simulink model "kalman"  (R2018b)
settings: Solver=VariableStepAuto  StartTime=0.0  StopTime=10.0  RelTol=1e-3
settings Model: Creator=axelwillekens  LastModifiedBy=axelwillekens

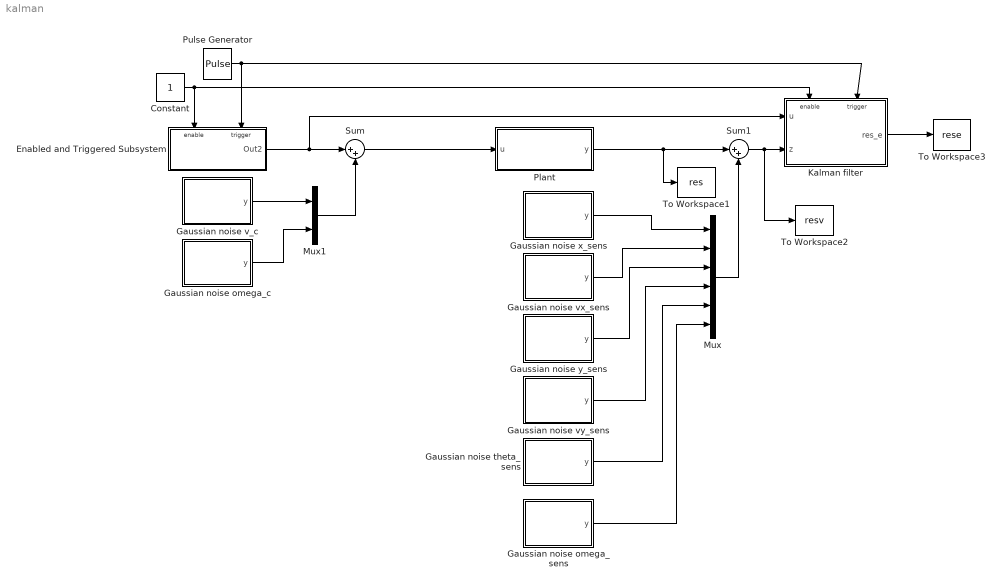
== system kalman ==
  Constant : Constant
  Enabled and Triggered Subsystem : Subsystem  TreatAsAtomicUnit=on
  Gaussian noise omega_c : MATLAB Function  TreatAsAtomicUnit=on
  Gaussian noise omega_sens : MATLAB Function  TreatAsAtomicUnit=on
  Gaussian noise theta_sens : MATLAB Function  TreatAsAtomicUnit=on
  Gaussian noise v_c : MATLAB Function  TreatAsAtomicUnit=on
  Gaussian noise vx_sens : MATLAB Function  TreatAsAtomicUnit=on
  Gaussian noise vy_sens : MATLAB Function  TreatAsAtomicUnit=on
  Gaussian noise x_sens : MATLAB Function  TreatAsAtomicUnit=on
  Gaussian noise y_sens : MATLAB Function  TreatAsAtomicUnit=on
  Kalman filter : Subsystem  TreatAsAtomicUnit=on
  Mux : Mux  Inputs=6
  Mux1 : Mux  Inputs=2
  Plant : Subsystem
  Pulse Generator : DiscretePulseGenerator  PulseType=Time based  Period=0.05  PulseWidth=5
  Sum : Sum  Inputs=|++
  Sum1 : Sum  Inputs=|++
  To Workspace1 : ToWorkspace  VariableName=res  SaveFormat=Timeseries  SampleTime=-1
  To Workspace2 : ToWorkspace  VariableName=resv  SaveFormat=Timeseries  SampleTime=-1
  To Workspace3 : ToWorkspace  VariableName=rese  SaveFormat=Timeseries  SampleTime=-1
  wires:
  Sum/1 -> Plant/1(u)
  Plant/1(y) -> To Workspace1/1, Sum1/1
  Sum1/1 -> To Workspace2/1, Kalman filter/2(z)
  Mux/1 -> Sum1/2
  Gaussian noise x_sens/1(y) -> Mux/1
  Gaussian noise vx_sens/1(y) -> Mux/2
  Gaussian noise y_sens/1(y) -> Mux/3
  Gaussian noise vy_sens/1(y) -> Mux/4
  Gaussian noise theta_sens/1(y) -> Mux/5
  Gaussian noise omega_sens/1(y) -> Mux/6
  Mux1/1 -> Sum/2
  Gaussian noise v_c/1(y) -> Mux1/1
  Gaussian noise omega_c/1(y) -> Mux1/2
  Enabled and Triggered Subsystem/1(Out2) -> Kalman filter/1(u), Sum/1
  Constant/1 -> Kalman filter/Enable, Enabled and Triggered Subsystem/Enable
  Pulse Generator/1 -> Enabled and Triggered Subsystem/Trigger, Kalman filter/Trigger
  Kalman filter/1(res_e) -> To Workspace3/1

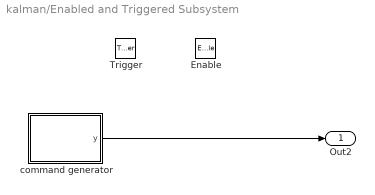
== system kalman/Enabled and Triggered Subsystem ==
  Enable : EnablePort
  Trigger : TriggerPort  VariantControl=Variant
  command generator : MATLAB Function  TreatAsAtomicUnit=on
  Out2 : Outport
  wires:
  command generator/1(y) -> Out2/1

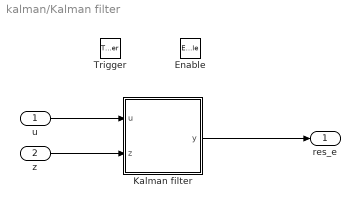
== system kalman/Kalman filter ==
  u : Inport
  z : Inport  Port=2
  Enable : EnablePort
  Trigger : TriggerPort  VariantControl=Variant
  Kalman filter : MATLAB Function  TreatAsAtomicUnit=on
  res_e : Outport
  wires:
  Kalman filter/1(y) -> res_e/1
  u/1 -> Kalman filter/1(u)
  z/1 -> Kalman filter/2(z)

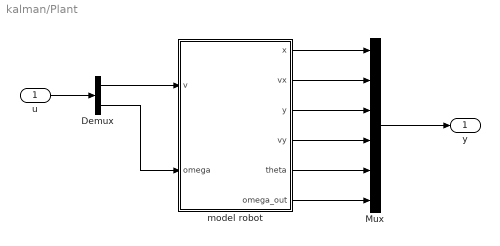
== system kalman/Plant ==
  u : Inport
  Demux : Demux  Outputs=2
  Mux : Mux  Inputs=6
  model robot : Subsystem
  y : Outport
  wires:
  Demux/1 -> model robot/1(v)
  Demux/2 -> model robot/2(omega)
  u/1 -> Demux/1
  model robot/1(x) -> Mux/1
  model robot/2(vx) -> Mux/2
  model robot/3(y) -> Mux/3
  model robot/4(vy) -> Mux/4
  model robot/5(theta) -> Mux/5
  model robot/6(omega_out) -> Mux/6
  Mux/1 -> y/1

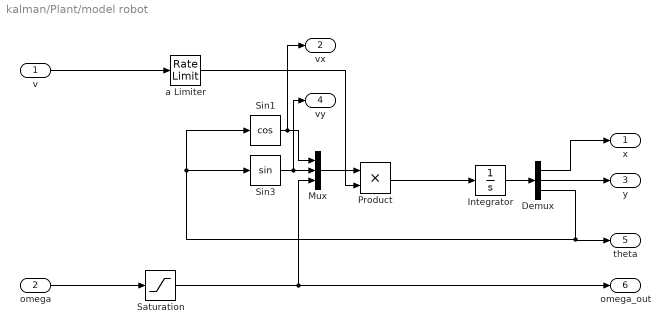
== system kalman/Plant/model robot ==
  v : Inport
  omega : Inport  Port=2
  Demux : Demux  Outputs=3
  Integrator : Integrator  InitialCondition=[2 -1 pi]
  Mux : Mux  Inputs=3
  Product : Product
  Saturation : Saturate  UpperLimit=50*(pi/180)  LowerLimit=-50*(pi/180)
  Sin1 : Trigonometry  Operator=cos
  Sin3 : Trigonometry
  a Limiter : RateLimiter  SampleTimeMode=inherited
  x : Outport
  vx : Outport  Port=2
  y : Outport  Port=3
  vy : Outport  Port=4
  theta : Outport  Port=5
  omega_out : Outport  Port=6
  wires:
  a Limiter/1 -> Product/2
  Mux/1 -> Product/1
  Product/1 -> Integrator/1
  Integrator/1 -> Demux/1
  Demux/2 -> y/1
  Demux/1 -> x/1
  Demux/3 -> Sin3/1, Sin1/1, theta/1
  Sin1/1 -> vx/1, Mux/1
  omega/1 -> Saturation/1
  Sin3/1 -> Mux/2, vy/1
  v/1 -> a Limiter/1
  Saturation/1 -> omega_out/1, Mux/3

== matlab function kalman/Gaussian noise theta_sens ==
  data: y output
function y = fcn()
standard_dev = 10.*(pi/180);
mu = 0;
y = standard_dev.*randn(1) + mu;

== matlab function kalman/Kalman filter/Kalman filter ==
  data: u input; y output; z input
function y = fcn(u,z)

persistent x P
%%%%%%%%%%%%%%%%%%%%%%%%%% initial conditions %%%%%%%%%%%%%%%%%%%%%%%%%%%%%
if isempty(x)
    % [x, vx, y, vy, theta, omega]
    x = [2; -1; -1; 0; pi; -0.8727];
end
if isempty(P)
    P = eye(6); % can't be zero, otherwise it will stay zero for ever!
end
theta_o = z(5);
Ts = 0.1;

%standard variations
varx = 0.02^2;
varvx = 0.1^2;
vary = 0.02^2;
varvy = 0.1^2;
vartheta = (10.*(pi/180))^2;
varomega = (4.*(pi/180))^2;

%%%%%%%%%%%%%%%%%%%%%%%%%%%%%%%%% the matrices %%%%%%%%%%%%%%%%%%%%%%%%%%%%
s.x = x;
s.P = P;
s.z = z;
s.u = u;
% A is F in text!!
s.A = [1 Ts 0 0 0 0;
        0 1 0 0 0 0;
        0 0 1 Ts 0 0;
        0 0 0 1 0 0;
        0 0 0 0 1 Ts;
        0 0 0 0 0 1];
s.B = [cos(theta_o)*Ts 0;
    cos(theta_o) 0;
    sin(theta_o)*Ts 0;
    sin(theta_o) 0;
    0 Ts;
    0 1];
s.H = eye(6);

s.R = [varx 0 0 0 0 0;
        0 varvx 0 0 0 0;
        0 0 vary 0 0 0;
        0 0 0 varvy 0 0;
        0 0 0 0 vartheta 0;
        0 0 0 0 0 varomega];
s.Q = eye(6);
%%%%%%%%%%%%%%%%%%%%%%%% calculate approximation of the next state%%%%%%%%%
ret = kalmanf(s);
x = ret.x;
P = ret.P;
y = x;

== matlab function kalman/Gaussian noise omega_sens ==
  data: y output
function y = fcn()
standard_dev = 4.*(pi/180);
mu = 0;
y = standard_dev.*randn(1) + mu;

== matlab function kalman/Gaussian noise vy_sens ==
  data: y output
function y = fcn()
standard_dev = 0.1;
mu = 0;
y = standard_dev.*randn(1) + mu;

== matlab function kalman/Gaussian noise vx_sens ==
  data: y output
function y = fcn()
standard_dev = 0.1;
mu = 0;
y = standard_dev.*randn(1) + mu;

== matlab function kalman/Gaussian noise y_sens ==
  data: y output
function y = fcn()
standard_dev = 0.08;
mu = 0;
y = standard_dev.*randn(1) + mu;

== matlab function kalman/Gaussian noise x_sens ==
  data: y output
function y = fcn()
standard_dev = 0.08;
mu = 0;
y = standard_dev.*randn(1) + mu;

== matlab function kalman/Gaussian noise v_c ==
  data: y output
function y = fcn()
standard_dev = 0.01;
mu = 0;
y = standard_dev.*randn(1) + mu;

== matlab function kalman/Gaussian noise omega_c ==
  data: y output
function y = fcn()
standard_dev = 0.01;
mu = 0;
y = standard_dev.*randn(1) + mu;

== matlab function kalman/Enabled and Triggered Subsystem/command generator ==
  data: y output
function y = fcn()
persistent i
if isempty(i)
    i = 1;
else
    i = i + 1;
end
a = [-0.8727
,-0.8727
,-0.8727
,-0.8727
,-0.8727
,-0.8727
,-0.8727
,-0.8727
,-0.8727
,-0.8727
,-0.8727
,-0.8727
,-0.8727
,-0.8727
,-0.8727
,-0.8727
,-0.8727
,-0.8727
,-0.8727
,-0.8727
,-0.8727
,-0.8727
,-0.8727
,-0.8727
,-0.8727
,-0.8727
,-0.8727
,-0.8727
,-0.8727
,-0.8727
,-0.6669
,-0.5229
,-0.4875
,-0.4649
,-0.4688
,-0.4645
,-0.4637
,-0.4632
,-0.4614
,-0.4566
,-0.4562
,-0.4545
,-0.4497
,-0.4493
,-0.4476
,-0.4428
,-0.4425
,-0.4408
,-0.4361
,-0.4357
,-0.4340
,-0.4294
,-0.4290
,-0.4274
,-0.4227
,-0.4224
,-0.4207
,-0.4162
,-0.4158
,-0.4142
,-0.4097
,-0.4094
,-0.4078
,-0.4033
,-0.4030
,-0.4014
,-0.3970
,-0.3966
,-0.3951
,-0.3907
,-0.3904
,-0.3889
,-0.3846
,-0.3843
,-0.3827
,-0.3785
,-0.3782
,-0.3767
,-0.3726
,-0.3723
,-0.3708
,-0.3667
,-0.3664
,-0.3650
,-0.3609
,-0.3607
,-0.3592
,-0.3553
,-0.3550
,-0.3536
,-0.3498
,-0.3495
,-0.3482
,-0.3444
,-0.3441
,-0.3428
,-0.3392
,-0.3389
,-0.3376
,-0.3341
,-0.3338
,-0.3325
,-0.3291
,-0.3289
,-0.3277
,-0.3243
,-0.3241
,-0.3229
,-0.3197
,-0.3195
,-0.3184
,-0.8727
,-0.8727
,-0.8727
,-0.8727
,-0.8727
,-0.8727
,-0.8727
,-0.8727
,-0.8727
,-0.8727
,-0.8727
,-0.8727
,-0.8727
,-0.8727
,-0.8727
,-0.8727
,-0.8727
,-0.8727
,-0.8727
,-0.8727
,-0.8727
,-0.8727
,-0.8727
,-0.8727
,-0.8727
,-0.8727
,-0.8727
,-0.8727
,-0.8727
,-0.8727
,-0.8727
,-0.8727
,-0.8727
,-0.8727
,-0.8727
,-0.8727
,-0.8727
,-0.8727
,-0.8727
,-0.8727
,-0.8727
,-0.8727
,-0.8727
,-0.8727
,-0.8727
,-0.8727
,-0.8727
,-0.8727
,-0.8727
,-0.8727
,-0.8727
,-0.8727
,-0.8727
,-0.8727
,-0.8727
,-0.8727
,-0.8727
,-0.8727
,-0.8727
,-0.8727
,-0.8727
,-0.8727
,-0.8727
,-0.8727
,-0.8727
,-0.8727
,-0.8727
,-0.8727
,-0.8727
,-0.8727
,-0.8727
,-0.8727
,-0.8727
,-0.8727
,-0.8727
,-0.8727
,-0.8727
,-0.8727
,-0.8727
,-0.8727
,-0.8727
,-0.8727
,-0.8727
,-0.8727
,-0.8727
,-0.8727
,-0.8727
,-0.8727
,-0.8727
,-0.8727
,-0.8727
,-0.8727
,-0.8727
,-0.8727
,-0.8727
,-0.8727
,-0.8727
,-0.8727
,-0.8727
,-0.8727
,-0.8727
,-0.8727
,-0.8727
,-0.8727
,-0.8727
,-0.8727
,0.8727
,0.8727
,0.8727
,0.8727
,0.8727
,0.8727
,0.8727
,0.8727
,0.8727
,0.8727
,0.0547
,-0.8727
,-0.8727
,-0.8727
,-0.8727
,-0.8727
,-0.8727
,-0.8727
,-0.8727
,-0.8727
,-0.8727
,-0.8727
,-0.8727
,-0.8727
,-0.8727
,-0.8727
,-0.8727
,-0.8727
,-0.8727
,-0.8727
,-0.8727
,-0.8727
,-0.8727
,-0.8727
,-0.8727
,-0.8727
,-0.8727
,-0.8727
,-0.8727
,-0.8727
,-0.8727
,-0.8727
,-0.8727
,-0.8727
,-0.8727
,-0.8727
,-0.8727
,-0.8727
,-0.8727
,-0.8727
,-0.8727
,-0.8727
,-0.8727
,-0.8727
,-0.8727
,-0.8727
,-0.8727
,-0.8727
,-0.8727
,-0.8727
,-0.8727
,-0.8727
,-0.8727
,-0.8484
,-0.8478
,-0.8403
,-0.8171
,-0.8155
,-0.8073
,-0.7844
,-0.7827
,-0.7745
,-0.7515
,-0.7498
,-0.7416
,-0.7185
,-0.7168
,-0.7085
,-0.6853
,-0.6836
,-0.6752
,-0.6518
,-0.6501
,-0.6416
,-0.6180
,-0.6162
,-0.6077
,-0.5838
,-0.5820
,-0.5733
,-0.5491
,-0.5473
,-0.5384
,-0.5138
,-0.5119
,-0.5029
,-0.4777
,-0.4758
,-0.4665
,-0.4407
,-0.4387
,-0.4292
,-0.4027
,-0.4006
,-0.3908
,-0.3633
,-0.3611
,-0.3509
,0.8727
,0.8727
,0.8727
,0.8727
,0.8727
,0.8727
,0.8727
,0.8727
,0.8727
,0.8727
,0.8727
,0.8727
,0.3583
,-0.1630
,-0.1690
,-0.1647
,-0.1637
,-0.1584
,-0.1431
,-0.1421
,-0.1367
,-0.1216
,-0.1205
,-0.1152
,-0.1003
,-0.0992
,-0.0939
,-0.0791
,-0.0781
,-0.0728
,-0.0582
,-0.0571
,-0.0519
,-0.0374
,-0.0363
,-0.0311
,-0.0167
,-0.0156
,-0.0105
,0.0039
,0.0049
,0.0101
,0.0243
,0.0254
,0.0305
,0.0447
,0.0458
,0.0509
,0.0651
,0.0661
,0.0712
,0.0854
,0.0864
,0.0915
,0.1057
,0.1068
,0.1119
,0.1261
,0.1271
,0.1323
,0.1465
,0.1476
,0.1528
,0.1671
,0.1682
,0.1734
,0.1879
,0.1890
,0.1942
,0.2088
,0.2099
,0.2153
,0.2301
,0.2312
,0.2366
,0.2516
,0.2528
,0.2583
,0.2736
,0.2748
,0.2804
,0.2960
,0.2972
,0.3030
,0.3190
,0.3203
,0.3262
,0.3427
,0.3440
,0.3501
,0.3672
,0.3685
,0.3748
,0.3925
,0.3939
,0.4005
,0.4189
,0.4204
,0.4272
,0.4465
,0.4481
,0.4553
,0.4756
,0.4772
,0.4849
,-0.8727
,-0.8727
,-0.8727
,-0.8727
,-0.8727
,-0.8727
,-0.8727
,-0.8727
,-0.8727
,-0.8727
,-0.8727
,-0.8727
,-0.8727
,-0.3570
,0.1071
,0.0609
,0.0660
,0.0668
,0.0699
,0.0783
,0.0789
,0.0819
,0.0902
,0.0908
,0.0938
,0.1021
,0.1027
,0.1056
,0.1138
,0.1144
,0.1173
,0.1254
,0.1260
,0.1289
,0.1370
,0.1376
,0.1405
,0.1485
,0.1491
,0.1520
,0.1600
,0.1606
,0.1635
,0.1715
,0.1721
,0.1749
,0.1829
,0.1835
,0.1864
,0.1944
,0.1950
,0.1979
,0.2060
,0.2066
,0.2095
,0.2176
,0.2182
,0.2211
,0.2293
,0.2299
,0.2329
,0.2411
,0.2418
,0.2448
,0.2532
,0.2538
,0.2568
,0.2654
,0.2660
,0.2691
,0.2778
,0.2785
,0.2817
,0.2906
,0.2913
,0.2945
,0.3037
,0.3044
,0.3077
,0.3172
,0.3179
,0.3214
,0.3312
,0.3319
,0.3355
,0.3457
,0.3465
,0.3503
,0.3609
,0.3617
,0.3657
,0.3768
,0.3777
,0.3819
,0.3937
,0.3946
,0.3990
,0.4115
,0.4125
,0.4172
,0.4306
,0.4317
,0.4367
,-0.8727
,-0.8727
,-0.8727
,-0.8727
,-0.8727
,-0.8727
,-0.8727
,-0.8727
,-0.8727
,-0.8727
,-0.8727
,-0.8727
,-0.8727
,-0.8727
,-0.8727
,-0.8727
,-0.4041
,-0.0089
,-0.0544
,-0.0592
,-0.0608
,-0.0553
,-0.0535
,-0.0528
,-0.0504
,-0.0442
,-0.0437
,-0.0414
,-0.0351
,-0.0347
,-0.0324
,-0.0262
,-0.0257
,-0.0235
,-0.0173
,-0.0168
,-0.0146
,-0.0084
,-0.0079
,-0.0057
,0.0005
,0.0010
,0.0032
,0.0094
,0.0099
,0.0121
,0.0183
,0.0188
,0.0211
,0.0273
,0.0278
,0.0300
,0.0363
,0.0368
,0.0390
,0.0454
,0.0458
,0.0481
,0.0545
,0.0550
,0.0573
,0.0638
,0.0643
,0.0667
,0.0732
,0.0737
,0.0761
,0.0829
,0.0834
,0.0858
,0.0927
,0.0932
,0.0957
,0.1028
,0.1033
,0.1059
,0.1131
,0.1137
,0.1164
,0.1239
,0.1245
,0.1272
,0.1350
,0.1356
,0.1385
,0.1467
,0.1473
,0.1503
,0.1589
,0.1596
,0.1628
,0.1718
,0.1725
,0.1759
,0.1855
,0.1863
,0.1899
,-0.8727
,-0.8727
,-0.8727
,-0.8727
,-0.8727
,-0.8727
,-0.8727
,-0.8727
,-0.8727
,-0.8727
,-0.8727
,-0.8727
,-0.8727
,-0.8727
,-0.8727
,-0.4337
,-0.0729
,-0.1305
,-0.1277
,-0.1241
,-0.1213
,-0.1190
,-0.1187
,-0.1168
,-0.1113
,-0.1110
,-0.1090
,-0.1037
,-0.1033
,-0.1013
,-0.0960
,-0.0956
,-0.0937
,-0.0884
,-0.0880
,-0.0861
,-0.0808
,-0.0804
,-0.0785
,-0.0732
,-0.0728
,-0.0710
,-0.0657
,-0.0653
,-0.0634
,-0.0581
,-0.0577
,-0.0558
,-0.0506
,-0.0502
,-0.0483
,-0.0430
,-0.0426
,-0.0407
,-0.0354
,-0.0350
,-0.0331
,-0.0277
,-0.0273
,-0.0254
,-0.0200
,-0.0196
,-0.0177
,-0.0122
,-0.0118
,-0.0098
,-0.0043
,-0.0039
,-0.0019
,0.0037
,0.0041
,0.0062
,0.0119
,0.0123
,0.0144
,0.0203
,0.0207
,0.0229
,0.0289
,0.0293
,0.0315
,0.0377
,0.0382
,0.0405
,0.0469
,0.0474
,0.0498
,0.0565
,0.0570
,0.0595
,0.0664
,0.0670
,0.0696
,0.0770
,0.0776
,0.0803
,0.0881
,0.0887
,0.0917
,-0.8727
,-0.8727
,-0.8727
,-0.8727
,-0.8727
,-0.8727
,-0.8727
,-0.8727
,-0.8727
,-0.8727
,-0.8727
,-0.8727
,-0.4380
,-0.0602
,-0.1093
,-0.1032
,-0.1027
,-0.1011
,-0.0967
,-0.0963
,-0.0948
,-0.0904
,-0.0900
,-0.0885
,-0.0841
,-0.0838
,-0.0822
,-0.0779
,-0.0775
,-0.0760
,-0.0717
,-0.0713
,-0.0698
,-0.0655
,-0.0652
,-0.0636
,-0.0593
,-0.0590
,-0.0575
,-0.0532
,-0.0529
,-0.0513
,-0.0470
,-0.0467
,-0.0452
,-0.0409
,-0.0406
,-0.0390
,-0.0347
,-0.0344
,-0.0328
,-0.0285
,-0.0282
,-0.0266
,-0.0223
,-0.0220
,-0.0204
,-0.0160
,-0.0157
,-0.0141
,-0.0097
,-0.0093
,-0.0077
,-0.0032
,-0.0029
,-0.0013
,0.0033
,0.0037
,0.0053
,0.0100
,0.0103
,0.0120
,0.0168
,0.0172
,0.0189
,0.0238
,0.0242
,0.0260
,0.0310
,0.0314
,0.0333
,0.0385
,0.0389
,0.0408
,0.0463
,0.0467
,0.0487
,0.0544
,0.0548
,0.0570
,0.0630
,0.0634
,0.0657
,0.0720
,0.0726
,0.0749
,-0.8727
,-0.8727
,-0.8727
,-0.8727
,-0.8727
,-0.8727
,-0.8727
,-0.8727
,-0.8727
,-0.8727
,-0.8727
,-0.3976
,-0.0042
,-0.0725
,-0.0607
,-0.0615
,-0.0611
,-0.0573
,-0.0571
,-0.0560
,-0.0526
,-0.0524
,-0.0512
,-0.0479
,-0.0476
,-0.0464
,-0.0431
,-0.0429
,-0.0417
,-0.0384
,-0.0382
,-0.0370
,-0.0337
,-0.0335
,-0.0323
,-0.0290
,-0.0288
,-0.0276
,-0.0243
,-0.0241
,-0.0229
,-0.0196
,-0.0194
,-0.0182
,-0.0149
,-0.0147
,-0.0135
,-0.0102
,-0.0100
,-0.0088
,-0.0055
,-0.0053
,-0.0041
,-0.0007
,-0.0005
,0.0007
,0.0041
,0.0043
,0.0055
,0.0089
,0.0092
,0.0104
,0.0139
,0.0141
,0.0154
,0.0189
,0.0192
,0.0205
,0.0240
,0.0243
,0.0256
,0.0293
,0.0296
,0.0309
,0.0347
,0.0350
,0.0364
,0.0403
,0.0406
,0.0420
,0.0461
,0.0464
,0.0479
,0.0521
,0.0524
,0.0540
,0.0584
,0.0588
,0.0604
,0.0651
,0.0655
,0.0672
,0.0722
,0.0726
,0.0745
,-0.8727
,-0.8727
,-0.8727
,-0.8727
,-0.8727
,-0.8727
,-0.8727
,-0.8727
,-0.8727
,-0.8727
,-0.4047
,0.0076
,-0.0420
,-0.0346
,-0.0356
,-0.0356
,-0.0327
,-0.0326
,-0.0318
,-0.0293
,-0.0291
,-0.0283
,-0.0258
,-0.0256
,-0.0248
,-0.0223
,-0.0222
,-0.0213
,-0.0189
,-0.0187
,-0.0178
,-0.0154
,-0.0152
,-0.0144
,-0.0119
,-0.0118
,-0.0109
,-0.0085
,-0.0083
,-0.0075
,-0.0050
,-0.0049
,-0.0040
,-0.0016
,-0.0014
,-0.0005
,0.0019
,0.0021
,0.0029
,0.0054
,0.0055
,0.0064
,0.0089
,0.0091
,0.0099
,0.0124
,0.0126
,0.0135
,0.0160
,0.0162
,0.0171
,0.0197
,0.0199
,0.0208
,0.0234
,0.0236
,0.0245
,0.0272
,0.0274
,0.0284
,0.0311
,0.0313
,0.0323
,0.0351
,0.0353
,0.0363
,0.0392
,0.0394
,0.0405
,0.0435
,0.0438
,0.0449
,0.0480
,0.0483
,0.0494
,0.0527
,0.0530
,0.0542
,0.0577
,0.0580
,0.0593
,0.0630
,0.0633
,0.0647
,-0.8727
,-0.8727
,-0.8727
,-0.8727
,-0.8727
,-0.8727
,-0.8727
,-0.8727
,-0.8727
,-0.4233
,-0.0003
,-0.0257
,-0.0235
,-0.0236
,-0.0232
,-0.0213
,-0.0212
,-0.0205
,-0.0187
,-0.0186
,-0.0180
,-0.0162
,-0.0160
,-0.0154
,-0.0136
,-0.0135
,-0.0129
,-0.0111
,-0.0110
,-0.0103
,-0.0086
,-0.0084
,-0.0078
,-0.0060
,-0.0059
,-0.0053
,-0.0035
,-0.0034
,-0.0028
,-0.0010
,-0.0009
,-0.0002
,0.0015
,0.0017
,0.0023
,0.0041
,0.0042
,0.0048
,0.0066
,0.0067
,0.0074
,0.0092
,0.0093
,0.0099
,0.0117
,0.0119
,0.0125
,0.0144
,0.0145
,0.0152
,0.0170
,0.0172
,0.0178
,0.0197
,0.0199
,0.0206
,0.0225
,0.0227
,0.0234
,0.0253
,0.0255
,0.0262
,0.0283
,0.0284
,0.0292
,0.0313
,0.0315
,0.0322
,0.0344
,0.0346
,0.0354
,0.0377
,0.0379
,0.0387
,0.0411
,0.0413
,0.0422
,0.0448
,0.0450
,0.0459
,0.0486
,0.0488
,0.0498
,-0.8727
,-0.8727
,-0.8727
,-0.8727
,-0.8727
,-0.8727
,-0.8727
,-0.8727
,-0.8727
,-0.3876
,0.0332
,-0.0232
,-0.0136
,-0.0155
,-0.0165
,-0.0144
,-0.0145
,-0.0142
,-0.0128
,-0.0127
,-0.0123
,-0.0110
,-0.0109
,-0.0104
,-0.0091
,-0.0090
,-0.0086
,-0.0073
,-0.0072
,-0.0067
,-0.0054
,-0.0054
,-0.0049
,-0.0036
,-0.0035
,-0.0031
,-0.0018
,-0.0017
,-0.0012
,0.0001
,0.0001
,0.0006
,0.0019
,0.0020
,0.0024
,0.0037
,0.0038
,0.0043
,0.0056
,0.0057
,0.0061
,0.0074
,0.0075
,0.0080
,0.0093
,0.0094
,0.0099
,0.0112
,0.0113
,0.0118
,0.0131
,0.0132
,0.0137
,0.0151
,0.0152
,0.0157
,0.0171
,0.0172
,0.0177
,0.0192
,0.0193
,0.0198
,0.0213
,0.0214
,0.0219
,0.0235
,0.0236
,0.0242
,0.0257
,0.0259
,0.0265
,0.0281
,0.0282
,0.0289
,0.0306
,0.0307
,0.0314
,0.0332
,0.0333
,0.0340
,0.0360
,0.0361
,0.0369
,0.0389
,0.0391
,0.0399
,-0.8727
,-0.8727
,-0.8727
,-0.8727
,-0.8727
,-0.8727
,-0.8727
,-0.8727
,-0.4252
,0.0047
,-0.0127
,-0.0118
,-0.0118
,-0.0116
,-0.0106
,-0.0105
,-0.0102
,-0.0092
,-0.0092
,-0.0088
,-0.0079
,-0.0078
,-0.0075
,-0.0065
,-0.0065
,-0.0061
,-0.0052
,-0.0051
,-0.0048
,-0.0038
,-0.0038
,-0.0034
,-0.0025
,-0.0024
,-0.0021
,-0.0012
,-0.0011
,-0.0008
,0.0002
,0.0003
,0.0006
,0.0015
,0.0016
,0.0019
,0.0029
,0.0029
,0.0033
,0.0042
,0.0043
,0.0046
,0.0056
,0.0057
,0.0060
,0.0070
,0.0071
,0.0074
,0.0084
,0.0085
,0.0088
,0.0098
,0.0099
,0.0103
,0.0113
,0.0114
,0.0117
,0.0128
,0.0128
,0.0132
,0.0143
,0.0144
,0.0148
,0.0159
,0.0160
,0.0164
,0.0175
,0.0176
,0.0180
,0.0192
,0.0193
,0.0197
,0.0210
,0.0211
,0.0216
,0.0229
,0.0230
,0.0235
,0.0249
,0.0250
,0.0255
,0.0270
,0.0271
,0.0277
,-0.8727
,-0.8727
,-0.8727
,-0.8727
,-0.8727
,-0.8727
,-0.3941
,0.0345
,-0.0110
,-0.0044
,-0.0059
,-0.0069
,-0.0056
,-0.0057
,-0.0056
,-0.0049
,-0.0049
,-0.0046
,-0.0039
,-0.0039
,-0.0037
,-0.0030
,-0.0029
,-0.0027
,-0.0020
,-0.0020
,-0.0018
,-0.0011
,-0.0010
,-0.0008
,-0.0001
,-0.0001
,0.0001
,0.0008
,0.0009
,0.0011
,0.0018
,0.0018
,0.0020
,0.0027
,0.0028
,0.0030
,0.0037
,0.0037
,0.0040
,0.0046
,0.0047
,0.0049
,0.0056
,0.0056
,0.0059
,0.0066
,0.0066
,0.0069
,0.0076
,0.0076
,0.0079
,0.0086
,0.0086
,0.0089
,0.0096
,0.0097
,0.0099
,0.0107
,0.0107
,0.0110
,0.0118
,0.0118
,0.0121
,0.0129
,0.0129
,0.0132
,0.0140
,0.0141
,0.0144
,0.0152
,0.0153
,0.0156
,0.0165
,0.0166
,0.0169
,0.0178
,0.0179
,0.0182
,0.0192
,0.0193
,0.0197
,0.0207
,0.0208
,0.0212
,-0.8727
,-0.8727
,-0.8727
,-0.8727
,-0.8727
,-0.4269
,0.0081
,-0.0030
,-0.0031
,-0.0028
,-0.0028
,-0.0027
,-0.0022
,-0.0022
,-0.0020
,-0.0016
,-0.0015
,-0.0014
,-0.0009
,-0.0009
,-0.0007
,-0.0003
,-0.0002
,-0.0001
,0.0004
,0.0004
,0.0006
,0.0010
,0.0011
,0.0012
,0.0017
,0.0017
,0.0019
,0.0023
,0.0024
,0.0025
,0.0030
,0.0030
,0.0032
,0.0036
,0.0037
,0.0038
,0.0043
,0.0043
,0.0045
,0.0049
,0.0050
,0.0051
,0.0056
,0.0056
,0.0058
,0.0063
,0.0063
,0.0065
,0.0070
,0.0070
,0.0072
,0.0076
,0.0077
,0.0079
,0.0083
,0.0084
,0.0086
,0.0091
,0.0091
,0.0093
,0.0098
,0.0099
,0.0100
,0.0106
,0.0106];

y = [1; a(i)];
